simulink model "Tractive_Motor_Ring_Four_Motors"  (R2020a)
settings: Solver=FixedStepDiscrete  StartTime=0.0  StopTime=10.0  FixedStep=0.001  RelTol=1e-3  EnableMultiTasking=on
PostLoadFcn:
  | , if any(exist('dsrtsu_mdlpostloadfcn', 'file') ~= 0), dsrtsu_mdlpostloadfcn('Execute', bdroot); end,
InitFcn:
  | , if any(exist('rtifpga_mdlclblib', 'file') ~= 0), rtifpga_mdlclblib('Init', bdroot); end,
undefined symbols (not defined in the file): RING_STATUS
settings Model: DSRTSU_INTERNAL_RTI_VER=560  DSRTSU_INTERNAL_RTI_TYPE=rti1401  RTICANMMDATA=struct('GeneralSetupData',struct('modelroot','C:\Users\harjo\Git\MACFormulaGit\MicroAutobox\rings\Tractive_Motor_Ring\Tractive_Motor_Ring_Four_Motors','generalsettings',struct('filesettings',struct('destfolder',struct('Name','RTICANMM_FILES','Check',1),'buildfolder',struct('Name','.','Check',1),'AbsDestfolder',struct('Name','C:\Users\harjo\Git\MACFormulaGit\MicroAutobox\rings\Tractive_Motor_Ring\Tractive_Motor_Ring_Four_Motors\RTICANMM_FILES'),'AbsBuildfolder',struct('Name','C:\Users\harjo\Git\MACFormulaGit\MicroAutobox\rings\Tractive_Motor_Ring\Tractive_Motor_Ring_Four_Motors'))),'options',struct('addpaths',1,'rmpaths',1,'addtrcexclusion',true,'cannavigator',struct('checkmonitoring',0),'show_usrtrc',0,'use_usrtrc',0),'advanced',struct('options',ones(1,100)),'MPSetup',{{}},'RTI',struct('Type','RTI1401','Ver','7.14','Date','02-May-2020'),'modelname','Tractive_Motor_Ring_Four_Motors','block','Tractive_Motor_Ring_Four_Motors'))  DSRTSU_INTERNAL_RTIFPGA=160  Creator=Harjot  LastModifiedBy=Harjot
settings DebuggingCC: SFUnexpectedBacktrackingDiag=warning  SFNoUnconditionalDefaultTransitionDiag=warning  SFExecutionAtInitializationDiag=none  ArithmeticOperatorsInVariantConditions=warning
settings HardwareCC: ProdBitPerPointer=32  ProdBitPerSizeT=32  ProdBitPerPtrDiffT=32  ProdLargestAtomicInteger=Integer  ProdEndianess=BigEndian  ProdWordSize=32  ProdHWDeviceType=Custom Processor->Custom  TargetIntDivRoundTo=Zero  TargetEndianess=BigEndian  TargetHWDeviceType=Custom Processor->Custom
settings SFSimCC: SimUseLocalCustomCode=off  MATLABDynamicMemAlloc=off  CustomCodeUndefinedFunction=UseInterfaceOnly
settings RTWCC: Description=dSPACE DS1401 Hardware Platform  SystemTargetFile=rti1401.tlc  MakeCommand=make_rti  TemplateMakefile=rti1401.tmf  RTWUseLocalCustomCode=off
settings CodeAppCC: StateflowObjectComments=on
settings STFCustomTargetCC: UtilityFuncGeneration=Shared location  ParMdlRefBuildCompliant=on  SystemTargetFile=rti1401.tlc
settings GRTTargetCC: TargetLangStandard=C89/C90 (ANSI)  UtilityFuncGeneration=Shared location  CompOptLevelCompliant=off  ConcurrentExecutionCompliant=off  CombineOutputUpdateFcns=off  MatFileLogging=off  CPPClassGenCompliant=off  UseToolchainInfoCompliant=off
settings ConfigComp: CovMetricSettings=dw  CovHtmlReporting=on  CovSaveCumulativeToWorkspaceVar=on  CovSaveSingleToWorkspaceVar=on  CovExternalEMLEnable=off

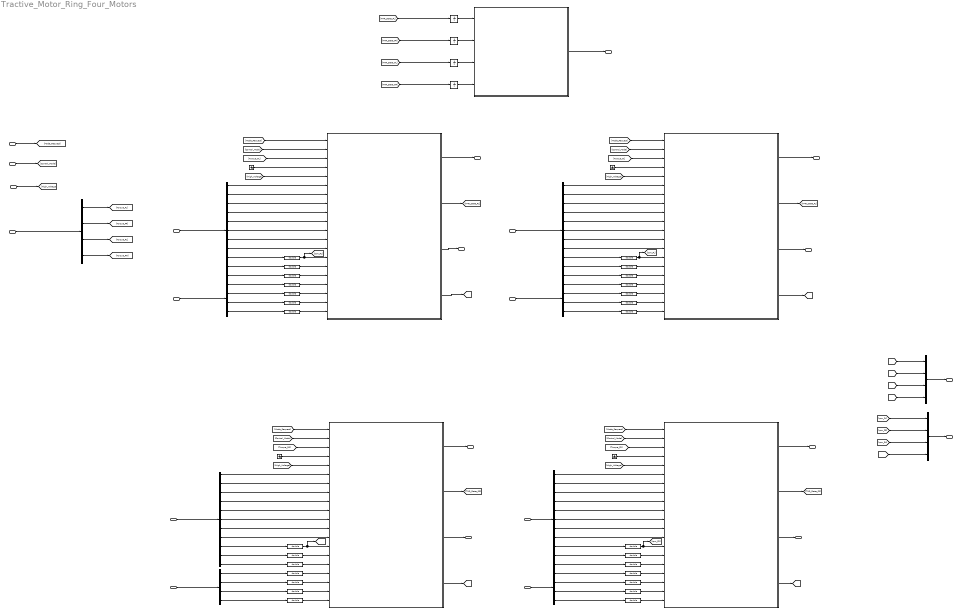
== system Tractive_Motor_Ring_Four_Motors ==
  MSR_Mode_Request : Inport  OutDataTypeStr=Enum: MSR_REQUEST
  Control_Mode : Inport  Port=2
  Accumulator_Voltage : Inport  Port=3
  Torque_Requests : Inport  Port=4  OutDataTypeStr=Bus: TorqueRequests
  Actual_Values1_FL : Inport  Port=5  OutDataTypeStr=Bus: AmkActualValues1
      settings: VarSizeSig=Yes
  Actual_Values1_FR : Inport  Port=6  OutDataTypeStr=Bus: AmkActualValues1
  Actual_Values1_RL : Inport  Port=7  OutDataTypeStr=Bus: AmkActualValues1
  Actual_Values1_RR : Inport  Port=8  OutDataTypeStr=Bus: AmkActualValues1
  Actual_Values2_FL : Inport  Port=9  OutDataTypeStr=Bus: AmkActualValues2
  Actual_Values2_FR : Inport  Port=10  OutDataTypeStr=Bus: AmkActualValues2
  Actual_Values2_RL : Inport  Port=11  OutDataTypeStr=Bus: AmkActualValues2
  Actual_Values2_RR : Inport  Port=12  OutDataTypeStr=Bus: AmkActualValues2
  Bus Creator : BusCreator  Inputs=4  OutDataTypeStr=Bus: TorqueLimits
      settings: InheritFromInputs=off
  Bus Creator1 : BusCreator  Inputs=4  OutDataTypeStr=Bus: MotorRPMs
      settings: InheritFromInputs=off
  Bus Selector : BusSelector  OutputSignals=TorqueFrontLeft,TorqueFrontRight,TorqueRearLeft,TorqueRearRight
  Bus Selector{1,3,5,7} (4 alike) : BusSelector  OutputSignals=AMK_bSystemReady,AMK_bError,AMK_bWarn,AMK_bQuitDcOn,AMK_bDcOn,AMK_bQuitInverterOn,AMK_bInverterOn,AMK_bDerating,AMK_ActualVelocity,AMK_TorqueCurrent,AMK_MagnetizingCurrent
  Bus Selector{2,4,6,8} (4 alike) : BusSelector  OutputSignals=AMK_TempMotor,AMK_TempInverter,AMK_ErrorInfo,AMK_TempIGBT
  Data Type Conversion{1..28} (28 alike) : DataTypeConversion  OutDataTypeStr=double
  Ground{,1..3} (4 alike) : Ground
  MasterTmr : Stateflow chart  TreatAsAtomicUnit=on
  TMR Front Left Motor : ModelReference  ModelNameDialog=Tractive_Motor_Ring_Single_Motor.slx  SimulationMode=Normal  ModelReferenceVersion=1.96
  TMR Front Right Motor : ModelReference  ModelNameDialog=Tractive_Motor_Ring_Single_Motor.slx  SimulationMode=Normal  ModelReferenceVersion=1.96
  TMR Rear Left Motor : ModelReference  ModelNameDialog=Tractive_Motor_Ring_Single_Motor.slx  SimulationMode=Normal  ModelReferenceVersion=1.96
  TMR Rear Right Motor : ModelReference  ModelNameDialog=Tractive_Motor_Ring_Single_Motor.slx  SimulationMode=Normal  ModelReferenceVersion=1.96
  Unit Delay{,1..3} (4 alike) : UnitDelay  InitialCondition=RING_STATUS.OFF  SampleTime=-1  HasFrameUpgradeWarning=on
  AMK_Setpoints_FL : Outport  OutDataTypeStr=Bus: AmkSetpoints  VectorParamsAs1DForOutWhenUnconnected=off
  AMK_Setpoints_FR : Outport  Port=2  OutDataTypeStr=Bus: AmkSetpoints  VectorParamsAs1DForOutWhenUnconnected=off
  AMK_Setpoints_RL : Outport  Port=3  OutDataTypeStr=Bus: AmkSetpoints  VectorParamsAs1DForOutWhenUnconnected=off
  AMK_Setpoints_RR : Outport  Port=4  OutDataTypeStr=Bus: AmkSetpoints  VectorParamsAs1DForOutWhenUnconnected=off
  Torque_Limits : Outport  Port=5  OutDataTypeStr=Bus: TorqueLimits  VectorParamsAs1DForOutWhenUnconnected=off
  TMR_State : Outport  Port=6  VectorParamsAs1DForOutWhenUnconnected=off
  Leaf_state_FL : Outport  Port=7  VectorParamsAs1DForOutWhenUnconnected=off
  Leaf_state_FR : Outport  Port=8  VectorParamsAs1DForOutWhenUnconnected=off
  Leaf_state_RL : Outport  Port=9  VectorParamsAs1DForOutWhenUnconnected=off
  Leaf_state_RR : Outport  Port=10  VectorParamsAs1DForOutWhenUnconnected=off
  MotorRpms : Outport  Port=11  OutDataTypeStr=Bus: MotorRPMs  VectorParamsAs1DForOutWhenUnconnected=off
  wires:
  Bus Selector7/11 -> Data Type Conversion10/1  "<AMK_MagnetizingCurrent>"
  Bus Selector7/2 -> TMR Rear Left Motor/7  "<AMK_bError>"
  Bus Selector1/10 -> Data Type Conversion6/1  "<AMK_TorqueCurrent>"
  Bus Selector7/6 -> TMR Rear Left Motor/11  "<AMK_bQuitInverterOn>"
  Bus Selector7/7 -> TMR Rear Left Motor/12  "<AMK_bInverterOn>"
  Bus Selector7/8 -> TMR Rear Left Motor/13  "<AMK_bDerating>"
  Bus Selector3/4 -> TMR Front Right Motor/9  "<AMK_bQuitDcOn>"
  Bus Selector7/3 -> TMR Rear Left Motor/8  "<AMK_bWarn>"
  Bus Selector7/9 -> Data Type Conversion11/1  "<AMK_ActualVelocity>"
  Bus Selector7/4 -> TMR Rear Left Motor/9  "<AMK_bQuitDcOn>"
  Bus Selector1/6 -> TMR Rear Right Motor/11  "<AMK_bQuitInverterOn>"
  Bus Selector2/4 -> Data Type Conversion21/1  "<AMK_TempIGBT>"
  [Control_Mode] -> TMR Front Right Motor/2
  Bus Selector3/11 -> Data Type Conversion4/1  "<AMK_MagnetizingCurrent>"
  [Torque_FL] -> TMR Front Left Motor/3
  Bus Selector/4 -> [Torque_RR]  "<TorqueRearRight>"
  Bus Selector1/5 -> TMR Rear Right Motor/10  "<AMK_bDcOn>"
  Actual_Values1_RL/1 -> Bus Selector7/1
  Bus Selector4/2 -> Data Type Conversion23/1  "<AMK_TempInverter>"
  Bus Selector3/10 -> Data Type Conversion3/1  "<AMK_TorqueCurrent>"
  Bus Selector3/7 -> TMR Front Right Motor/12  "<AMK_bInverterOn>"
  Bus Selector2/2 -> Data Type Conversion20/1  "<AMK_TempInverter>"
  Bus Selector3/3 -> TMR Front Right Motor/8  "<AMK_bWarn>"
  Bus Selector3/6 -> TMR Front Right Motor/11  "<AMK_bQuitInverterOn>"
  Bus Selector1/3 -> TMR Rear Right Motor/8  "<AMK_bWarn>"
  Bus Selector/2 -> [Torque_FR]  "<TorqueFrontRight>"
  Bus Selector3/5 -> TMR Front Right Motor/10  "<AMK_bDcOn>"
  Bus Selector2/1 -> Data Type Conversion19/1  "<AMK_TempMotor>"
  [Control_Mode] -> TMR Front Left Motor/2
  Bus Selector1/11 -> Data Type Conversion7/1  "<AMK_MagnetizingCurrent>"
  Bus Selector2/3 -> Data Type Conversion27/1  "<AMK_ErrorInfo>"
  Bus Selector3/8 -> TMR Front Right Motor/13  "<AMK_bDerating>"
  Bus Selector3/9 -> Data Type Conversion5/1  "<AMK_ActualVelocity>"
  Bus Selector3/2 -> TMR Front Right Motor/7  "<AMK_bError>"
  Actual_Values2_RL/1 -> Bus Selector8/1
  Bus Selector3/1 -> TMR Front Right Motor/6  "<AMK_bSystemReady>"
  Bus Selector1/9 -> Data Type Conversion8/1  "<AMK_ActualVelocity>"
  Bus Selector1/1 -> TMR Rear Right Motor/6  "<AMK_bSystemReady>"
  Actual_Values1_RR/1 -> Bus Selector1/1
  [Mode_Request] -> TMR Rear Right Motor/1
  [High_Voltage] -> TMR Front Left Motor/5
  [High_Voltage] -> TMR Rear Right Motor/5
  [Mode_Request] -> TMR Front Right Motor/1
  [Mode_Request] -> TMR Front Left Motor/1
  [Torque_FR] -> TMR Front Right Motor/3
  Bus Selector1/4 -> TMR Rear Right Motor/9  "<AMK_bQuitDcOn>"
  Actual_Values2_FR/1 -> Bus Selector4/1
  [High_Voltage] -> TMR Front Right Motor/5
  [Torque_RR] -> TMR Rear Right Motor/3
  [Control_Mode] -> TMR Rear Right Motor/2
  Torque_Requests/1 -> Bus Selector/1
  Accumulator_Voltage/1 -> [High_Voltage]
  Bus Selector4/3 -> Data Type Conversion26/1  "<AMK_ErrorInfo>"
  Control_Mode/1 -> [Control_Mode]
  Bus Selector4/4 -> Data Type Conversion24/1  "<AMK_TempIGBT>"
  Bus Selector/1 -> [Torque_FL]  "<TorqueFrontLeft>"
  Bus Selector4/1 -> Data Type Conversion22/1  "<AMK_TempMotor>"
  Actual_Values2_FL/1 -> Bus Selector6/1
  TMR Front Left Motor/3 -> Leaf_state_FL/1
  Ground/1 -> TMR Rear Right Motor/4
  TMR Rear Left Motor/2 -> [TMR_State_RL]
  TMR Front Left Motor/2 -> [TMR_State_FL]
  Ground2/1 -> TMR Front Left Motor/4
  Bus Selector8/3 -> Data Type Conversion28/1  "<AMK_ErrorInfo>"
  Bus Selector8/4 -> Data Type Conversion18/1  "<AMK_TempIGBT>"
  TMR Rear Right Motor/2 -> [TMR_State_RR]
  [Mode_Request] -> TMR Rear Left Motor/1
  TMR Front Right Motor/2 -> [TMR_State_FR]
  Ground1/1 -> TMR Front Right Motor/4
  TMR Front Right Motor/4 -> [TL_FR]
  [TL_FR] -> Bus Creator/2  "TorqueLimitFrontRight"
  TMR Front Left Motor/1 -> AMK_Setpoints_FL/1
  [TL_RL] -> Bus Creator/3  "TorqueLimitRearLeft"
  [TL_FL] -> Bus Creator/1  "TorqueLimitFrontLeft"
  Bus Selector1/7 -> TMR Rear Right Motor/12  "<AMK_bInverterOn>"
  Bus Selector1/8 -> TMR Rear Right Motor/13  "<AMK_bDerating>"
  Bus Selector/3 -> [Torque_RL]  "<TorqueRearLeft>"
  Bus Selector1/2 -> TMR Rear Right Motor/7  "<AMK_bError>"
  TMR Rear Left Motor/4 -> [TL_RL]
  TMR Front Left Motor/4 -> [TL_FL]
  [Control_Mode] -> TMR Rear Left Motor/2
  Bus Selector7/1 -> TMR Rear Left Motor/6  "<AMK_bSystemReady>"
  [High_Voltage] -> TMR Rear Left Motor/5
  Bus Selector8/2 -> Data Type Conversion17/1  "<AMK_TempInverter>"
  Actual_Values1_FL/1 -> Bus Selector5/1
  Actual_Values2_RR/1 -> Bus Selector2/1
  TMR Rear Right Motor/4 -> [TL_RR]
  TMR Rear Left Motor/3 -> Leaf_state_RL/1
  MSR_Mode_Request/1 -> [Mode_Request]
  Bus Selector8/1 -> Data Type Conversion16/1  "<AMK_TempMotor>"
  Bus Selector7/5 -> TMR Rear Left Motor/10  "<AMK_bDcOn>"
  Bus Creator/1 -> Torque_Limits/1
  TMR Front Right Motor/3 -> Leaf_state_FR/1
  TMR Rear Right Motor/3 -> Leaf_state_RR/1
  [Torque_RL] -> TMR Rear Left Motor/3
  Actual_Values1_FR/1 -> Bus Selector3/1
  [TL_RR] -> Bus Creator/4  "TorqueLimitRearRight"
  Bus Selector7/10 -> Data Type Conversion9/1  "<AMK_TorqueCurrent>"
  Ground3/1 -> TMR Rear Left Motor/4
  Bus Selector5/1 -> TMR Front Left Motor/6  "<AMK_bSystemReady>"
  Bus Selector5/2 -> TMR Front Left Motor/7  "<AMK_bError>"
  Bus Selector5/3 -> TMR Front Left Motor/8  "<AMK_bWarn>"
  Bus Selector5/4 -> TMR Front Left Motor/9  "<AMK_bQuitDcOn>"
  Bus Selector5/5 -> TMR Front Left Motor/10  "<AMK_bDcOn>"
  Bus Selector5/6 -> TMR Front Left Motor/11  "<AMK_bQuitInverterOn>"
  Bus Selector5/7 -> TMR Front Left Motor/12  "<AMK_bInverterOn>"
  Bus Selector5/8 -> TMR Front Left Motor/13  "<AMK_bDerating>"
  Bus Selector5/9 -> Data Type Conversion2/1  "<AMK_ActualVelocity>"
  Bus Selector5/10 -> Data Type Conversion1/1  "<AMK_TorqueCurrent>"
  Bus Selector5/11 -> Data Type Conversion12/1  "<AMK_MagnetizingCurrent>"
  Bus Selector6/1 -> Data Type Conversion13/1  "<AMK_TempMotor>"
  Bus Selector6/2 -> Data Type Conversion14/1  "<AMK_TempInverter>"
  Bus Selector6/3 -> Data Type Conversion25/1  "<AMK_ErrorInfo>"
  Bus Selector6/4 -> Data Type Conversion15/1  "<AMK_TempIGBT>"
  TMR Front Right Motor/1 -> AMK_Setpoints_FR/1
  TMR Rear Right Motor/1 -> AMK_Setpoints_RR/1
  TMR Rear Left Motor/1 -> AMK_Setpoints_RL/1
  [TMR_State_FL] -> Unit Delay/1  "TmrStatusFl"
  [TMR_State_FR] -> Unit Delay1/1  "TmrStatusFr"
  [TMR_State_RR] -> Unit Delay3/1  "TmrStatusRr"
  [TMR_State_RL] -> Unit Delay2/1  "TmrStatusRl"
  MasterTmr/1(TmrState) -> TMR_State/1
  Unit Delay/1 -> MasterTmr/1(TmrStatusFl)
  Unit Delay1/1 -> MasterTmr/2(TmrStatusFr)
  Unit Delay2/1 -> MasterTmr/3(TmrStatusRl)
  Unit Delay3/1 -> MasterTmr/4(TmrStatusRr)
  Data Type Conversion12/1 -> TMR Front Left Motor/16
  Data Type Conversion1/1 -> TMR Front Left Motor/15
  Data Type Conversion3/1 -> TMR Front Right Motor/15
  Data Type Conversion4/1 -> TMR Front Right Motor/16
  Data Type Conversion7/1 -> TMR Rear Right Motor/16
  Data Type Conversion6/1 -> TMR Rear Right Motor/15
  Data Type Conversion9/1 -> TMR Rear Left Motor/15
  Data Type Conversion10/1 -> TMR Rear Left Motor/16
  Data Type Conversion13/1 -> TMR Front Left Motor/17
  Data Type Conversion15/1 -> TMR Front Left Motor/20
  Data Type Conversion18/1 -> TMR Rear Left Motor/20
  Data Type Conversion16/1 -> TMR Rear Left Motor/17
  Data Type Conversion19/1 -> TMR Rear Right Motor/17
  Data Type Conversion21/1 -> TMR Rear Right Motor/20
  Data Type Conversion22/1 -> TMR Front Right Motor/17
  Data Type Conversion24/1 -> TMR Front Right Motor/20
  Data Type Conversion23/1 -> TMR Front Right Motor/18
  Data Type Conversion20/1 -> TMR Rear Right Motor/18
  Data Type Conversion14/1 -> TMR Front Left Motor/18
  Data Type Conversion17/1 -> TMR Rear Left Motor/18
  Data Type Conversion25/1 -> TMR Front Left Motor/19
  Data Type Conversion26/1 -> TMR Front Right Motor/19
  Data Type Conversion27/1 -> TMR Rear Right Motor/19
  Data Type Conversion28/1 -> TMR Rear Left Motor/19
  Bus Creator1/1 -> MotorRpms/1
  Data Type Conversion11/1 -> TMR Rear Left Motor/14, [rpm_RL]
  Data Type Conversion2/1 -> TMR Front Left Motor/14, [rpm_FL]
  Data Type Conversion5/1 -> TMR Front Right Motor/14, [rpm_FR]
  Data Type Conversion8/1 -> TMR Rear Right Motor/14, [rpm_RR]
  [rpm_FL] -> Bus Creator1/1  "RpmFrontLeft"
  [rpm_FR] -> Bus Creator1/2  "RpmFrontRight"
  [rpm_RL] -> Bus Creator1/3  "RpmRearLeft"
  [rpm_RR] -> Bus Creator1/4  "RpmRearRight"

== stateflow chart Tractive_Motor_Ring_Four_Motors/MasterTmr ==
  state SHUTDOWN
    entry:
    TmrState = RING_STATUS.SHUTDOWN_COMPLETE_HV;
  state OFF
    entry:
    TmrState = RING_STATUS.OFF;
  state STARTUP_LV
    entry:
    TmrState = RING_STATUS.STARTUP_COMPLETE_LV;
  state RUNNING
    entry:
    TmrState = RING_STATUS.RUNNING;
  state STARTUP_HV1
    entry:
    TmrState = RING_STATUS.STARTUP_COMPLETE_HV;
  (default) -> OFF
  OFF -> STARTUP_LV : [TmrStatusFl == RING_STATUS.STARTUP_COMPLETE_LV && ...
      | TmrStatusFr == RING_STATUS.STARTUP_COMPLETE_LV && ...
      | TmrStatusRl == RING_STATUS.STARTUP_COMPLETE_LV && ...
      | TmrStatusRr == RING_STATUS.STARTUP_COMPLETE_LV]
  RUNNING -> SHUTDOWN : [TmrStatusFl == RING_STATUS.SHUTDOWN_COMPLETE_HV && ...
      | TmrStatusFr == RING_STATUS.SHUTDOWN_COMPLETE_HV && ...
      | TmrStatusRl == RING_STATUS.SHUTDOWN_COMPLETE_HV && ...
      | TmrStatusRr == RING_STATUS.SHUTDOWN_COMPLETE_HV]
  STARTUP_HV1 -> RUNNING : [TmrStatusFl == RING_STATUS.RUNNING && ...
      | TmrStatusFr == RING_STATUS.RUNNING && ...
      | TmrStatusRl == RING_STATUS.RUNNING && ...
      | TmrStatusRr == RING_STATUS.RUNNING]
  STARTUP_LV -> STARTUP_HV1 : [TmrStatusFl == RING_STATUS.STARTUP_COMPLETE_HV && ...
      | TmrStatusFr == RING_STATUS.STARTUP_COMPLETE_HV && ...
      | TmrStatusRl == RING_STATUS.STARTUP_COMPLETE_HV && ...
      | TmrStatusRr == RING_STATUS.STARTUP_COMPLETE_HV]
  data: TmrStatusFl input Enum: RING_STATUS; TmrStatusFr input Enum: RING_STATUS; TmrStatusRl input Enum: RING_STATUS; TmrStatusRr input Enum: RING_STATUS; TmrState output Enum: RING_STATUS =RING_STATUS.OFF
